simulink model "Previous_Version_2016_b_All_BPF_with_IQ_Demodulation"  (R2020a)
settings: Solver=VariableStepAuto  StartTime=0.0  StopTime=8.2  RelTol=1e-3
libraries: dsphdlxfrm x1
(part 1 of 3)
settings Model: Creator=Renas  LastModifiedBy=Renas

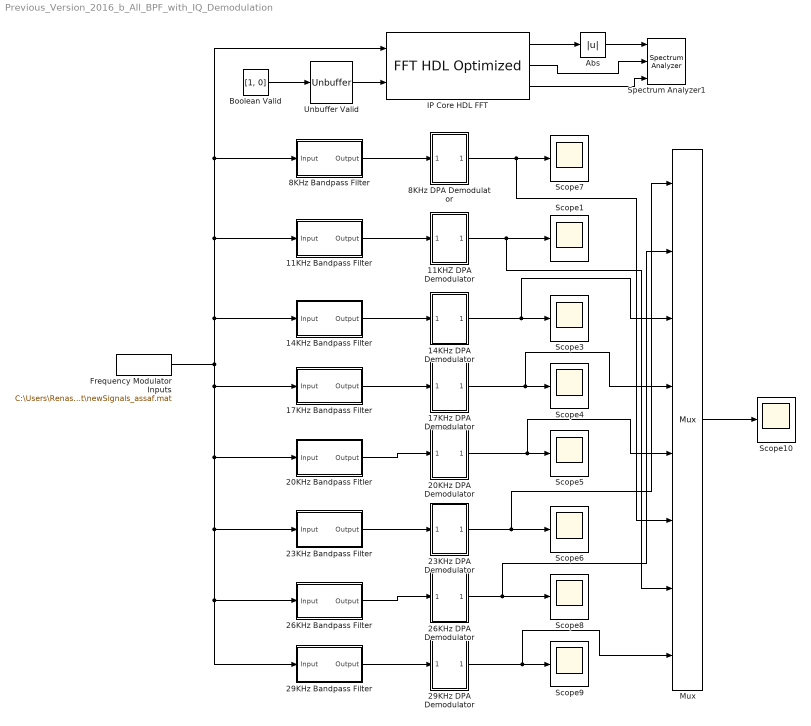
== system Previous_Version_2016_b_All_BPF_with_IQ_Demodulation ==
  11KHZ DPA Demodulator : Subsystem
  11KHz Bandpass Filter : Subsystem  Tag=FilterWizardSubSystem
      settings: ErrorFcn=dspFilterRealizedInBasicElemsAlgLoopErrFcnCallback
  14KHz Bandpass Filter : Subsystem  Tag=FilterWizardSubSystem
      settings: ErrorFcn=dspFilterRealizedInBasicElemsAlgLoopErrFcnCallback
  14KHz DPA Demodulator : Subsystem
  17KHz Bandpass Filter : Subsystem  Tag=FilterWizardSubSystem
      settings: ErrorFcn=dspFilterRealizedInBasicElemsAlgLoopErrFcnCallback
  17KHz DPA Demodulator : Subsystem
  20KHz Bandpass Fitler : Subsystem  Tag=FilterWizardSubSystem
      settings: ErrorFcn=dspFilterRealizedInBasicElemsAlgLoopErrFcnCallback
  20KHz DPA Demodulator : Subsystem
  23KHz Bandpass Filter : Subsystem  Tag=FilterWizardSubSystem
      settings: ErrorFcn=dspFilterRealizedInBasicElemsAlgLoopErrFcnCallback
  23KHz DPA Demodulator : Subsystem
  26KHz Bandpass Filter : Subsystem  Tag=FilterWizardSubSystem
      settings: ErrorFcn=dspFilterRealizedInBasicElemsAlgLoopErrFcnCallback
  26KHz DPA Demodulator : Subsystem
  29KHz Bandpass Filter : Subsystem  Tag=FilterWizardSubSystem
      settings: ErrorFcn=dspFilterRealizedInBasicElemsAlgLoopErrFcnCallback
  29KHz DPA Demodulator : Subsystem
  8KHz Bandpass Filter : Subsystem  Tag=FilterWizardSubSystem
      settings: ErrorFcn=dspFilterRealizedInBasicElemsAlgLoopErrFcnCallback
  8KHz DPA Demodulator : Subsystem
  Abs : Abs
  Boolean Valid : Constant  Value=[1, 0]  OutDataTypeStr=boolean  SampleTime=0.000004
  Frequency Modulator Inputs : FromFile  FileName=C:\Users\Renas\Desktop\Final Year Project\newSignals_assaf.mat  SampleTime=0.000004
  IP Core HDL FFT : dsphdlxfrm/FFT HDL Optimized  FFTLength=8  Architecture=Burst Radix 2  ComplexMultiplication=Use 4 multipliers and 2 adders  BitReversedOutput=off  BitReversedInput=off  Normalize=off  SimulateUsing=Code generation  RoundingMethod=Nearest  ResetInputPort=off  StartOutputPort=off  EndOutputPort=off
      settings: SourceProductBaseCode=DS
  Mux : Mux  Inputs=8
      settings: DisplayOption=signals
  Scope{1,3..10} (9 alike) : Scope
  Spectrum Analyzer1 : SpectrumAnalyzer  NumInputPorts=3
  Unbuffer Valid : Unbuffer
  wires:
  8KHz Bandpass Filter/1(Output) -> 8KHz DPA Demodulator/1(In3)
  11KHZ DPA Demodulator/1(Out1) -> Mux/7, Scope1/1
  11KHz Bandpass Filter/1(Output) -> 11KHZ DPA Demodulator/1(Output)
  14KHz DPA Demodulator/1(Out1) -> Mux/3, Scope3/1
  17KHz DPA Demodulator/1(Out1) -> Scope4/1, Mux/4
  20KHz DPA Demodulator/1(Out1) -> Scope5/1, Mux/5
  23KHz DPA Demodulator/1(Out1) -> Mux/1, Scope6/1
  26KHz DPA Demodulator/1(Out1) -> Mux/2, Scope8/1
  29KHz DPA Demodulator/1(Out1) -> Mux/8, Scope9/1
  Mux/1 -> Scope10/1
  8KHz DPA Demodulator/1(Out1) -> Mux/6, Scope7/1
  14KHz Bandpass Filter/1(Output) -> 14KHz DPA Demodulator/1(Output)
  17KHz Bandpass Filter/1(Output) -> 17KHz DPA Demodulator/1(Output)
  20KHz Bandpass Fitler/1(Output) -> 20KHz DPA Demodulator/1(Output)
  23KHz Bandpass Filter/1(Output) -> 23KHz DPA Demodulator/1(Output)
  26KHz Bandpass Filter/1(Output) -> 26KHz DPA Demodulator/1(Output)
  29KHz Bandpass Filter/1(Output) -> 29KHz DPA Demodulator/1(Output)
  Frequency Modulator Inputs/1 -> IP Core HDL FFT/1, 8KHz Bandpass Filter/1(Input), 11KHz Bandpass Filter/1(Input), 14KHz Bandpass Filter/1(Input), 29KHz Bandpass Filter/1(Input), 26KHz Bandpass Filter/1(Input), 23KHz Bandpass Filter/1(Input), 20KHz Bandpass Fitler/1(Input), 17KHz Bandpass Filter/1(Input)
  IP Core HDL FFT/1 -> Abs/1
  IP Core HDL FFT/3 -> Spectrum Analyzer1/3
  IP Core HDL FFT/2 -> Spectrum Analyzer1/2
  Abs/1 -> Spectrum Analyzer1/1
  Boolean Valid/1 -> Unbuffer Valid/1
  Unbuffer Valid/1 -> IP Core HDL FFT/2

== system Previous_Version_2016_b_All_BPF_with_IQ_Demodulation/11KHZ DPA Demodulator ==
  note: "Imaginary"
  note: "Real"
  Output : Inport
  Delay : Delay  DelayLength=1  InitialCondition=0
  Delay1 : Delay  DelayLength=1  InitialCondition=0
  Divide : Product  Inputs=*/
  Gain1 : Gain  Gain=7.5/((0.000004)*(2*pi*1000))
  Gain2 : Gain  Gain=-1
  LPF_11000Hz_Elliptical_100dB_BW_2KHz_Order_1 : Subsystem  Tag=FilterWizardSubSystem
      settings: ErrorFcn=dspFilterRealizedInBasicElemsAlgLoopErrFcnCallback
  LPF_11000Hz_Elliptical_100dB_BW_2KHz_Order_10 : Subsystem  Tag=FilterWizardSubSystem
      settings: ErrorFcn=dspFilterRealizedInBasicElemsAlgLoopErrFcnCallback
  Product{5..10} (6 alike) : Product
  Scope : Scope
  Scope5 : Scope
  Scope6 : Scope
  Sine Wave : Sin  Frequency=2*pi*11000  Phase=+(pi/2)  Samples=250  SampleTime=1/250000
  Sine Wave1 : Sin  Frequency=2*pi*11000  SampleTime=1/250000
  Sum : Sum  Inputs=|++
  Sum1 : Sum  Inputs=|+-
  Trigonometric Function1 : Trigonometry  Operator=atan
  Out1 : Outport
  wires:
  LPF_11000Hz_Elliptical_100dB_BW_2KHz_Order_10/1(Output) -> Scope5/1, Product10/1, Product9/1, Delay1/1
  Delay/1 -> Product8/1, Product9/2
  Gain2/1 -> Product8/2, Product6/2, Delay/1
  Delay1/1 -> Product6/1, Product10/2
  Divide/1 -> Trigonometric Function1/1
  Gain1/1 -> Out1/1
  Product6/1 -> Sum1/1
  Sum/1 -> Divide/2
  Sum1/1 -> Divide/1
  Product5/1 -> LPF_11000Hz_Elliptical_100dB_BW_2KHz_Order_10/1(Input)
  Product8/1 -> Sum/2
  Product9/1 -> Sum1/2
  Sine Wave1/1 -> Product5/2
  Output/1 -> Product5/1, Product7/2, Scope/1
  LPF_11000Hz_Elliptical_100dB_BW_2KHz_Order_1/1(Output) -> Gain2/1, Scope6/1
  Product10/1 -> Sum/1
  Sine Wave/1 -> Product7/1
  Product7/1 -> LPF_11000Hz_Elliptical_100dB_BW_2KHz_Order_1/1(Input)
  Trigonometric Function1/1 -> Gain1/1

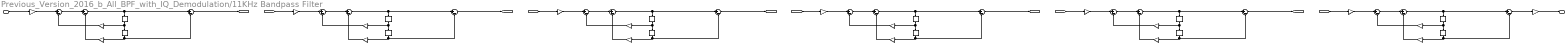
== system Previous_Version_2016_b_All_BPF_with_IQ_Demodulation/11KHz Bandpass Filter ==
  Input : Inport
  Delay{11..16,21..26} (12 alike) : Delay  DelayLength=1  InitialCondition=0
  SumA{21..26,31..36} (12 alike) : Sum  Inputs=|+-  RndMeth=Nearest  SaturateOnIntegerOverflow=on  OutDataTypeStr=Inherit: Same as first input
  SumB{31..36} (6 alike) : Sum  Inputs=|+-  RndMeth=Nearest  SaturateOnIntegerOverflow=on  OutDataTypeStr=Inherit: Same as first input
  a(2)(1) : Gain  Gain=-1.9065952938784374  ParamDataTypeStr=double  RndMeth=Nearest  SaturateOnIntegerOverflow=on  OutDataTypeStr=Inherit: Same as input
  a(2)(2) : Gain  Gain=-1.93433571126361903  ParamDataTypeStr=double  RndMeth=Nearest  SaturateOnIntegerOverflow=on  OutDataTypeStr=Inherit: Same as input
  a(2)(3) : Gain  Gain=-1.90539970784921886  ParamDataTypeStr=double  RndMeth=Nearest  SaturateOnIntegerOverflow=on  OutDataTypeStr=Inherit: Same as input
  a(2)(4) : Gain  Gain=-1.92628834700168183  ParamDataTypeStr=double  RndMeth=Nearest  SaturateOnIntegerOverflow=on  OutDataTypeStr=Inherit: Same as input
  a(2)(5) : Gain  Gain=-1.90953396328044223  ParamDataTypeStr=double  RndMeth=Nearest  SaturateOnIntegerOverflow=on  OutDataTypeStr=Inherit: Same as input
  a(2)(6) : Gain  Gain=-1.91729782266235227  ParamDataTypeStr=double  RndMeth=Nearest  SaturateOnIntegerOverflow=on  OutDataTypeStr=Inherit: Same as input
  a(3)(1) : Gain  Gain=0.996606493218230471  ParamDataTypeStr=double  RndMeth=Nearest  SaturateOnIntegerOverflow=on  OutDataTypeStr=Inherit: Same as input
  a(3)(2) : Gain  Gain=0.997154789899552862  ParamDataTypeStr=double  RndMeth=Nearest  SaturateOnIntegerOverflow=on  OutDataTypeStr=Inherit: Same as input
  a(3)(3) : Gain  Gain=0.990951691511379074  ParamDataTypeStr=double  RndMeth=Nearest  SaturateOnIntegerOverflow=on  OutDataTypeStr=Inherit: Same as input
  a(3)(4) : Gain  Gain=0.992044936946816946  ParamDataTypeStr=double  RndMeth=Nearest  SaturateOnIntegerOverflow=on  OutDataTypeStr=Inherit: Same as input
  a(3)(5) : Gain  Gain=0.988127915993850081  ParamDataTypeStr=double  RndMeth=Nearest  SaturateOnIntegerOverflow=on  OutDataTypeStr=Inherit: Same as input
  a(3)(6) : Gain  Gain=0.98867412178745806  ParamDataTypeStr=double  RndMeth=Nearest  SaturateOnIntegerOverflow=on  OutDataTypeStr=Inherit: Same as input
  s(1) : Gain  Gain=0.0249744654943324963  ParamDataTypeStr=double  RndMeth=Nearest  SaturateOnIntegerOverflow=on  OutDataTypeStr=Inherit: Same as input
  s(2) : Gain  Gain=0.0249744654943324963  ParamDataTypeStr=double  RndMeth=Nearest  SaturateOnIntegerOverflow=on  OutDataTypeStr=Inherit: Same as input
  s(3) : Gain  Gain=0.0186903150291070699  ParamDataTypeStr=double  RndMeth=Nearest  SaturateOnIntegerOverflow=on  OutDataTypeStr=Inherit: Same as input
  s(4) : Gain  Gain=0.0186903150291070699  ParamDataTypeStr=double  RndMeth=Nearest  SaturateOnIntegerOverflow=on  OutDataTypeStr=Inherit: Same as input
  s(5) : Gain  Gain=0.00882552998553000692  ParamDataTypeStr=double  RndMeth=Nearest  SaturateOnIntegerOverflow=on  OutDataTypeStr=Inherit: Same as input
  s(6) : Gain  Gain=0.00882552998553000692  ParamDataTypeStr=double  RndMeth=Nearest  SaturateOnIntegerOverflow=on  OutDataTypeStr=Inherit: Same as input
  s(7) : Gain  Gain=0.891250938133745563  ParamDataTypeStr=double  RndMeth=Nearest  SaturateOnIntegerOverflow=on  OutDataTypeStr=Inherit: Same as input
  Output : Outport
  wires:
  Input/1 -> s(1)/1
  s(1)/1 -> SumA21/1
  SumA21/1 -> SumA31/1
  SumA31/1 -> SumB31/1, Delay11/1
  SumB31/1 -> [Sect1]
  a(2)(1)/1 -> SumA21/2
  Delay11/1 -> a(2)(1)/1, Delay21/1
  a(3)(1)/1 -> SumA31/2
  Delay21/1 -> a(3)(1)/1, SumB31/2
  [Sect1] -> s(2)/1
  s(2)/1 -> SumA22/1
  SumA22/1 -> SumA32/1
  SumA32/1 -> SumB32/1, Delay12/1
  SumB32/1 -> [Sect2]
  a(2)(2)/1 -> SumA22/2
  Delay12/1 -> a(2)(2)/1, Delay22/1
  a(3)(2)/1 -> SumA32/2
  Delay22/1 -> a(3)(2)/1, SumB32/2
  [Sect2] -> s(3)/1
  s(3)/1 -> SumA23/1
  SumA23/1 -> SumA33/1
  SumA33/1 -> SumB33/1, Delay13/1
  SumB33/1 -> [Sect3]
  a(2)(3)/1 -> SumA23/2
  Delay13/1 -> a(2)(3)/1, Delay23/1
  a(3)(3)/1 -> SumA33/2
  Delay23/1 -> a(3)(3)/1, SumB33/2
  [Sect3] -> s(4)/1
  s(4)/1 -> SumA24/1
  SumA24/1 -> SumA34/1
  SumA34/1 -> SumB34/1, Delay14/1
  SumB34/1 -> [Sect4]
  a(2)(4)/1 -> SumA24/2
  Delay14/1 -> a(2)(4)/1, Delay24/1
  a(3)(4)/1 -> SumA34/2
  Delay24/1 -> a(3)(4)/1, SumB34/2
  [Sect4] -> s(5)/1
  s(5)/1 -> SumA25/1
  SumA25/1 -> SumA35/1
  SumA35/1 -> SumB35/1, Delay15/1
  SumB35/1 -> [Sect5]
  a(2)(5)/1 -> SumA25/2
  Delay15/1 -> a(2)(5)/1, Delay25/1
  a(3)(5)/1 -> SumA35/2
  Delay25/1 -> a(3)(5)/1, SumB35/2
  [Sect5] -> s(6)/1
  s(6)/1 -> SumA26/1
  SumA26/1 -> SumA36/1
  SumA36/1 -> SumB36/1, Delay16/1
  SumB36/1 -> s(7)/1
  a(2)(6)/1 -> SumA26/2
  Delay16/1 -> a(2)(6)/1, Delay26/1
  a(3)(6)/1 -> SumA36/2
  Delay26/1 -> a(3)(6)/1, SumB36/2
  s(7)/1 -> Output/1

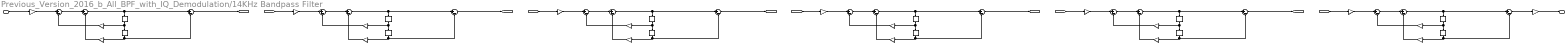
== system Previous_Version_2016_b_All_BPF_with_IQ_Demodulation/14KHz Bandpass Filter ==
  Input : Inport
  Delay{11..16,21..26} (12 alike) : Delay  DelayLength=1  InitialCondition=0
  SumA{21..26,31..36} (12 alike) : Sum  Inputs=|+-  RndMeth=Nearest  SaturateOnIntegerOverflow=on  OutDataTypeStr=Inherit: Same as first input
  SumB{31..36} (6 alike) : Sum  Inputs=|+-  RndMeth=Nearest  SaturateOnIntegerOverflow=on  OutDataTypeStr=Inherit: Same as first input
  a(2)(1) : Gain  Gain=-1.85547628075388515  ParamDataTypeStr=double  RndMeth=Nearest  SaturateOnIntegerOverflow=on  OutDataTypeStr=Inherit: Same as input
  a(2)(2) : Gain  Gain=-1.89037409301842607  ParamDataTypeStr=double  RndMeth=Nearest  SaturateOnIntegerOverflow=on  OutDataTypeStr=Inherit: Same as input
  a(2)(3) : Gain  Gain=-1.85544003350902065  ParamDataTypeStr=double  RndMeth=Nearest  SaturateOnIntegerOverflow=on  OutDataTypeStr=Inherit: Same as input
  a(2)(4) : Gain  Gain=-1.88139619531860136  ParamDataTypeStr=double  RndMeth=Nearest  SaturateOnIntegerOverflow=on  OutDataTypeStr=Inherit: Same as input
  a(2)(5) : Gain  Gain=-1.86125831898491256  ParamDataTypeStr=double  RndMeth=Nearest  SaturateOnIntegerOverflow=on  OutDataTypeStr=Inherit: Same as input
  a(2)(6) : Gain  Gain=-1.87084185582867502  ParamDataTypeStr=double  RndMeth=Nearest  SaturateOnIntegerOverflow=on  OutDataTypeStr=Inherit: Same as input
  a(3)(1) : Gain  Gain=0.996669751260965242  ParamDataTypeStr=double  RndMeth=Nearest  SaturateOnIntegerOverflow=on  OutDataTypeStr=Inherit: Same as input
  a(3)(2) : Gain  Gain=0.997091501071703412  ParamDataTypeStr=double  RndMeth=Nearest  SaturateOnIntegerOverflow=on  OutDataTypeStr=Inherit: Same as input
  a(3)(3) : Gain  Gain=0.991078116538709697  ParamDataTypeStr=double  RndMeth=Nearest  SaturateOnIntegerOverflow=on  OutDataTypeStr=Inherit: Same as input
  a(3)(4) : Gain  Gain=0.991918388588846511  ParamDataTypeStr=double  RndMeth=Nearest  SaturateOnIntegerOverflow=on  OutDataTypeStr=Inherit: Same as input
  a(3)(5) : Gain  Gain=0.988191259658187882  ParamDataTypeStr=double  RndMeth=Nearest  SaturateOnIntegerOverflow=on  OutDataTypeStr=Inherit: Same as input
  a(3)(6) : Gain  Gain=0.988610747171366766  ParamDataTypeStr=double  RndMeth=Nearest  SaturateOnIntegerOverflow=on  OutDataTypeStr=Inherit: Same as input
  s(1) : Gain  Gain=0.0249744654943327288  ParamDataTypeStr=double  RndMeth=Nearest  SaturateOnIntegerOverflow=on  OutDataTypeStr=Inherit: Same as input
  s(2) : Gain  Gain=0.0249744654943327288  ParamDataTypeStr=double  RndMeth=Nearest  SaturateOnIntegerOverflow=on  OutDataTypeStr=Inherit: Same as input
  s(3) : Gain  Gain=0.0186903150291072434  ParamDataTypeStr=double  RndMeth=Nearest  SaturateOnIntegerOverflow=on  OutDataTypeStr=Inherit: Same as input
  s(4) : Gain  Gain=0.0186903150291072434  ParamDataTypeStr=double  RndMeth=Nearest  SaturateOnIntegerOverflow=on  OutDataTypeStr=Inherit: Same as input
  s(5) : Gain  Gain=0.00882552998553009019  ParamDataTypeStr=double  RndMeth=Nearest  SaturateOnIntegerOverflow=on  OutDataTypeStr=Inherit: Same as input
  s(6) : Gain  Gain=0.00882552998553009019  ParamDataTypeStr=double  RndMeth=Nearest  SaturateOnIntegerOverflow=on  OutDataTypeStr=Inherit: Same as input
  s(7) : Gain  Gain=0.891250938133745563  ParamDataTypeStr=double  RndMeth=Nearest  SaturateOnIntegerOverflow=on  OutDataTypeStr=Inherit: Same as input
  Output : Outport
  wires:
  Input/1 -> s(1)/1
  s(1)/1 -> SumA21/1
  SumA21/1 -> SumA31/1
  SumA31/1 -> SumB31/1, Delay11/1
  SumB31/1 -> [Sect1]
  a(2)(1)/1 -> SumA21/2
  Delay11/1 -> a(2)(1)/1, Delay21/1
  a(3)(1)/1 -> SumA31/2
  Delay21/1 -> a(3)(1)/1, SumB31/2
  [Sect1] -> s(2)/1
  s(2)/1 -> SumA22/1
  SumA22/1 -> SumA32/1
  SumA32/1 -> SumB32/1, Delay12/1
  SumB32/1 -> [Sect2]
  a(2)(2)/1 -> SumA22/2
  Delay12/1 -> a(2)(2)/1, Delay22/1
  a(3)(2)/1 -> SumA32/2
  Delay22/1 -> a(3)(2)/1, SumB32/2
  [Sect2] -> s(3)/1
  s(3)/1 -> SumA23/1
  SumA23/1 -> SumA33/1
  SumA33/1 -> SumB33/1, Delay13/1
  SumB33/1 -> [Sect3]
  a(2)(3)/1 -> SumA23/2
  Delay13/1 -> a(2)(3)/1, Delay23/1
  a(3)(3)/1 -> SumA33/2
  Delay23/1 -> a(3)(3)/1, SumB33/2
  [Sect3] -> s(4)/1
  s(4)/1 -> SumA24/1
  SumA24/1 -> SumA34/1
  SumA34/1 -> SumB34/1, Delay14/1
  SumB34/1 -> [Sect4]
  a(2)(4)/1 -> SumA24/2
  Delay14/1 -> a(2)(4)/1, Delay24/1
  a(3)(4)/1 -> SumA34/2
  Delay24/1 -> a(3)(4)/1, SumB34/2
  [Sect4] -> s(5)/1
  s(5)/1 -> SumA25/1
  SumA25/1 -> SumA35/1
  SumA35/1 -> SumB35/1, Delay15/1
  SumB35/1 -> [Sect5]
  a(2)(5)/1 -> SumA25/2
  Delay15/1 -> a(2)(5)/1, Delay25/1
  a(3)(5)/1 -> SumA35/2
  Delay25/1 -> a(3)(5)/1, SumB35/2
  [Sect5] -> s(6)/1
  s(6)/1 -> SumA26/1
  SumA26/1 -> SumA36/1
  SumA36/1 -> SumB36/1, Delay16/1
  SumB36/1 -> s(7)/1
  a(2)(6)/1 -> SumA26/2
  Delay16/1 -> a(2)(6)/1, Delay26/1
  a(3)(6)/1 -> SumA36/2
  Delay26/1 -> a(3)(6)/1, SumB36/2
  s(7)/1 -> Output/1

== system Previous_Version_2016_b_All_BPF_with_IQ_Demodulation/14KHz DPA Demodulator ==
  note: "Imaginary"
  note: "Real"
  Output : Inport
  Delay : Delay  DelayLength=1  InitialCondition=0
  Delay1 : Delay  DelayLength=1  InitialCondition=0
  Divide : Product  Inputs=*/
  Gain1 : Gain  Gain=7.5/((0.000004)*(2*pi*1000))
  Gain2 : Gain  Gain=-1
  LPF_14060Hz_Elliptical_100dB_BW_2KHz_Order_1 : Subsystem  Tag=FilterWizardSubSystem
      settings: ErrorFcn=dspFilterRealizedInBasicElemsAlgLoopErrFcnCallback
  LPF_14060Hz_Elliptical_100dB_BW_2KHz_Order_10 : Subsystem  Tag=FilterWizardSubSystem
      settings: ErrorFcn=dspFilterRealizedInBasicElemsAlgLoopErrFcnCallback
  Product{5..10} (6 alike) : Product
  Scope : Scope
  Scope5 : Scope
  Scope6 : Scope
  Sine Wave : Sin  Frequency=2*pi*14060  Phase=+(pi/2)  Samples=250  SampleTime=1/250000
  Sine Wave1 : Sin  Frequency=2*pi*14060  SampleTime=1/250000
  Sum : Sum  Inputs=|++
  Sum1 : Sum  Inputs=|+-
  Trigonometric Function1 : Trigonometry  Operator=atan
  Out1 : Outport
  wires:
  LPF_14060Hz_Elliptical_100dB_BW_2KHz_Order_10/1(Output) -> Scope5/1, Product10/1, Product9/1, Delay1/1
  Delay/1 -> Product8/1, Product9/2
  Gain2/1 -> Product8/2, Product6/2, Delay/1
  Delay1/1 -> Product6/1, Product10/2
  Divide/1 -> Trigonometric Function1/1
  Gain1/1 -> Out1/1
  Product6/1 -> Sum1/1
  Sum/1 -> Divide/2
  Sum1/1 -> Divide/1
  Product5/1 -> LPF_14060Hz_Elliptical_100dB_BW_2KHz_Order_10/1(Input)
  Product8/1 -> Sum/2
  Product9/1 -> Sum1/2
  Sine Wave1/1 -> Product5/2
  Output/1 -> Product5/1, Product7/2, Scope/1
  LPF_14060Hz_Elliptical_100dB_BW_2KHz_Order_1/1(Output) -> Gain2/1, Scope6/1
  Product10/1 -> Sum/1
  Sine Wave/1 -> Product7/1
  Product7/1 -> LPF_14060Hz_Elliptical_100dB_BW_2KHz_Order_1/1(Input)
  Trigonometric Function1/1 -> Gain1/1

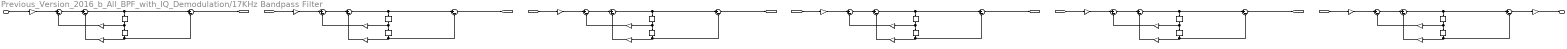
== system Previous_Version_2016_b_All_BPF_with_IQ_Demodulation/17KHz Bandpass Filter ==
  Input : Inport
  Delay{11..16,21..26} (12 alike) : Delay  DelayLength=1  InitialCondition=0
  SumA{21..26,31..36} (12 alike) : Sum  Inputs=|+-  RndMeth=Nearest  SaturateOnIntegerOverflow=on  OutDataTypeStr=Inherit: Same as first input
  SumB{31..36} (6 alike) : Sum  Inputs=|+-  RndMeth=Nearest  SaturateOnIntegerOverflow=on  OutDataTypeStr=Inherit: Same as first input
  a(2)(1) : Gain  Gain=-1.79490617474365566  ParamDataTypeStr=double  RndMeth=Nearest  SaturateOnIntegerOverflow=on  OutDataTypeStr=Inherit: Same as input
  a(2)(2) : Gain  Gain=-1.83664366102072707  ParamDataTypeStr=double  RndMeth=Nearest  SaturateOnIntegerOverflow=on  OutDataTypeStr=Inherit: Same as input
  a(2)(3) : Gain  Gain=-1.79598178570065503  ParamDataTypeStr=double  RndMeth=Nearest  SaturateOnIntegerOverflow=on  OutDataTypeStr=Inherit: Same as input
  a(2)(4) : Gain  Gain=-1.82682896191897925  ParamDataTypeStr=double  RndMeth=Nearest  SaturateOnIntegerOverflow=on  OutDataTypeStr=Inherit: Same as input
  a(2)(5) : Gain  Gain=-1.80343450281448359  ParamDataTypeStr=double  RndMeth=Nearest  SaturateOnIntegerOverflow=on  OutDataTypeStr=Inherit: Same as input
  a(2)(6) : Gain  Gain=-1.81478470631303734  ParamDataTypeStr=double  RndMeth=Nearest  SaturateOnIntegerOverflow=on  OutDataTypeStr=Inherit: Same as input
  a(3)(1) : Gain  Gain=0.996710356003254083  ParamDataTypeStr=double  RndMeth=Nearest  SaturateOnIntegerOverflow=on  OutDataTypeStr=Inherit: Same as input
  a(3)(2) : Gain  Gain=0.997050880802035189  ParamDataTypeStr=double  RndMeth=Nearest  SaturateOnIntegerOverflow=on  OutDataTypeStr=Inherit: Same as input
  a(3)(3) : Gain  Gain=0.991159132334594517  ParamDataTypeStr=double  RndMeth=Nearest  SaturateOnIntegerOverflow=on  OutDataTypeStr=Inherit: Same as input
  a(3)(4) : Gain  Gain=0.991837310732544997  ParamDataTypeStr=double  RndMeth=Nearest  SaturateOnIntegerOverflow=on  OutDataTypeStr=Inherit: Same as input
  a(3)(5) : Gain  Gain=0.988231779244872266  ParamDataTypeStr=double  RndMeth=Nearest  SaturateOnIntegerOverflow=on  OutDataTypeStr=Inherit: Same as input
  a(3)(6) : Gain  Gain=0.988570212046192665  ParamDataTypeStr=double  RndMeth=Nearest  SaturateOnIntegerOverflow=on  OutDataTypeStr=Inherit: Same as input
  s(1) : Gain  Gain=0.0249744654943329404  ParamDataTypeStr=double  RndMeth=Nearest  SaturateOnIntegerOverflow=on  OutDataTypeStr=Inherit: Same as input
  s(2) : Gain  Gain=0.0249744654943329404  ParamDataTypeStr=double  RndMeth=Nearest  SaturateOnIntegerOverflow=on  OutDataTypeStr=Inherit: Same as input
  s(3) : Gain  Gain=0.018690315029107403  ParamDataTypeStr=double  RndMeth=Nearest  SaturateOnIntegerOverflow=on  OutDataTypeStr=Inherit: Same as input
  s(4) : Gain  Gain=0.018690315029107403  ParamDataTypeStr=double  RndMeth=Nearest  SaturateOnIntegerOverflow=on  OutDataTypeStr=Inherit: Same as input
  s(5) : Gain  Gain=0.00882552998553016305  ParamDataTypeStr=double  RndMeth=Nearest  SaturateOnIntegerOverflow=on  OutDataTypeStr=Inherit: Same as input
  s(6) : Gain  Gain=0.00882552998553016305  ParamDataTypeStr=double  RndMeth=Nearest  SaturateOnIntegerOverflow=on  OutDataTypeStr=Inherit: Same as input
  s(7) : Gain  Gain=0.891250938133745563  ParamDataTypeStr=double  RndMeth=Nearest  SaturateOnIntegerOverflow=on  OutDataTypeStr=Inherit: Same as input
  Output : Outport
  wires:
  Input/1 -> s(1)/1
  s(1)/1 -> SumA21/1
  SumA21/1 -> SumA31/1
  SumA31/1 -> SumB31/1, Delay11/1
  SumB31/1 -> [Sect1]
  a(2)(1)/1 -> SumA21/2
  Delay11/1 -> a(2)(1)/1, Delay21/1
  a(3)(1)/1 -> SumA31/2
  Delay21/1 -> a(3)(1)/1, SumB31/2
  [Sect1] -> s(2)/1
  s(2)/1 -> SumA22/1
  SumA22/1 -> SumA32/1
  SumA32/1 -> SumB32/1, Delay12/1
  SumB32/1 -> [Sect2]
  a(2)(2)/1 -> SumA22/2
  Delay12/1 -> a(2)(2)/1, Delay22/1
  a(3)(2)/1 -> SumA32/2
  Delay22/1 -> a(3)(2)/1, SumB32/2
  [Sect2] -> s(3)/1
  s(3)/1 -> SumA23/1
  SumA23/1 -> SumA33/1
  SumA33/1 -> SumB33/1, Delay13/1
  SumB33/1 -> [Sect3]
  a(2)(3)/1 -> SumA23/2
  Delay13/1 -> a(2)(3)/1, Delay23/1
  a(3)(3)/1 -> SumA33/2
  Delay23/1 -> a(3)(3)/1, SumB33/2
  [Sect3] -> s(4)/1
  s(4)/1 -> SumA24/1
  SumA24/1 -> SumA34/1
  SumA34/1 -> SumB34/1, Delay14/1
  SumB34/1 -> [Sect4]
  a(2)(4)/1 -> SumA24/2
  Delay14/1 -> a(2)(4)/1, Delay24/1
  a(3)(4)/1 -> SumA34/2
  Delay24/1 -> a(3)(4)/1, SumB34/2
  [Sect4] -> s(5)/1
  s(5)/1 -> SumA25/1
  SumA25/1 -> SumA35/1
  SumA35/1 -> SumB35/1, Delay15/1
  SumB35/1 -> [Sect5]
  a(2)(5)/1 -> SumA25/2
  Delay15/1 -> a(2)(5)/1, Delay25/1
  a(3)(5)/1 -> SumA35/2
  Delay25/1 -> a(3)(5)/1, SumB35/2
  [Sect5] -> s(6)/1
  s(6)/1 -> SumA26/1
  SumA26/1 -> SumA36/1
  SumA36/1 -> SumB36/1, Delay16/1
  SumB36/1 -> s(7)/1
  a(2)(6)/1 -> SumA26/2
  Delay16/1 -> a(2)(6)/1, Delay26/1
  a(3)(6)/1 -> SumA36/2
  Delay26/1 -> a(3)(6)/1, SumB36/2
  s(7)/1 -> Output/1

== system Previous_Version_2016_b_All_BPF_with_IQ_Demodulation/17KHz DPA Demodulator ==
  note: "Imaginary"
  note: "Real"
  Output : Inport
  Delay : Delay  DelayLength=1  InitialCondition=0
  Delay1 : Delay  DelayLength=1  InitialCondition=0
  Divide : Product  Inputs=*/
  Gain1 : Gain  Gain=7.5/((0.000004)*(2*pi*1000))
  Gain2 : Gain  Gain=-1
  LPF_17050Hz_Elliptical_100dB_BW_2KHz_Order_1 : Subsystem  Tag=FilterWizardSubSystem
      settings: ErrorFcn=dspFilterRealizedInBasicElemsAlgLoopErrFcnCallback
  LPF_17050Hz_Elliptical_100dB_BW_2KHz_Order_10 : Subsystem  Tag=FilterWizardSubSystem
      settings: ErrorFcn=dspFilterRealizedInBasicElemsAlgLoopErrFcnCallback
  Product{5..10} (6 alike) : Product
  Scope : Scope
  Scope5 : Scope
  Scope6 : Scope
  Sine Wave : Sin  Frequency=2*pi*17050  Phase=+(pi/2)  Samples=250  SampleTime=1/250000
  Sine Wave1 : Sin  Frequency=2*pi*17050  SampleTime=1/250000
  Sum : Sum  Inputs=|++
  Sum1 : Sum  Inputs=|+-
  Trigonometric Function1 : Trigonometry  Operator=atan
  Out1 : Outport
  wires:
  LPF_17050Hz_Elliptical_100dB_BW_2KHz_Order_10/1(Output) -> Scope5/1, Product10/1, Product9/1, Delay1/1
  Delay/1 -> Product8/1, Product9/2
  Gain2/1 -> Product8/2, Product6/2, Delay/1
  Delay1/1 -> Product6/1, Product10/2
  Divide/1 -> Trigonometric Function1/1
  Gain1/1 -> Out1/1
  Product6/1 -> Sum1/1
  Sum/1 -> Divide/2
  Sum1/1 -> Divide/1
  Product5/1 -> LPF_17050Hz_Elliptical_100dB_BW_2KHz_Order_10/1(Input)
  Product8/1 -> Sum/2
  Product9/1 -> Sum1/2
  Sine Wave1/1 -> Product5/2
  Output/1 -> Product5/1, Product7/2, Scope/1
  LPF_17050Hz_Elliptical_100dB_BW_2KHz_Order_1/1(Output) -> Gain2/1, Scope6/1
  Product10/1 -> Sum/1
  Sine Wave/1 -> Product7/1
  Product7/1 -> LPF_17050Hz_Elliptical_100dB_BW_2KHz_Order_1/1(Input)
  Trigonometric Function1/1 -> Gain1/1

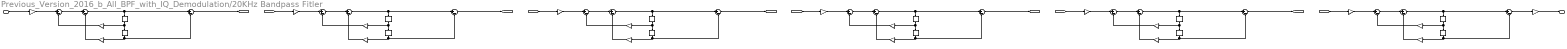
== system Previous_Version_2016_b_All_BPF_with_IQ_Demodulation/20KHz Bandpass Fitler ==
  Input : Inport
  Delay{11..16,21..26} (12 alike) : Delay  DelayLength=1  InitialCondition=0
  SumA{21..26,31..36} (12 alike) : Sum  Inputs=|+-  RndMeth=Nearest  SaturateOnIntegerOverflow=on  OutDataTypeStr=Inherit: Same as first input
  SumB{31..36} (6 alike) : Sum  Inputs=|+-  RndMeth=Nearest  SaturateOnIntegerOverflow=on  OutDataTypeStr=Inherit: Same as first input
  a(2)(1) : Gain  Gain=-1.72621306906651273  ParamDataTypeStr=double  RndMeth=Nearest  SaturateOnIntegerOverflow=on  OutDataTypeStr=Inherit: Same as input
  a(2)(2) : Gain  Gain=-1.77440557550816225  ParamDataTypeStr=double  RndMeth=Nearest  SaturateOnIntegerOverflow=on  OutDataTypeStr=Inherit: Same as input
  a(2)(3) : Gain  Gain=-1.72835364533195657  ParamDataTypeStr=double  RndMeth=Nearest  SaturateOnIntegerOverflow=on  OutDataTypeStr=Inherit: Same as input
  a(2)(4) : Gain  Gain=-1.76384098848158066  ParamDataTypeStr=double  RndMeth=Nearest  SaturateOnIntegerOverflow=on  OutDataTypeStr=Inherit: Same as input
  a(2)(5) : Gain  Gain=-1.73736864335266916  ParamDataTypeStr=double  RndMeth=Nearest  SaturateOnIntegerOverflow=on  OutDataTypeStr=Inherit: Same as input
  a(2)(6) : Gain  Gain=-1.75039999440418348  ParamDataTypeStr=double  RndMeth=Nearest  SaturateOnIntegerOverflow=on  OutDataTypeStr=Inherit: Same as input
  a(3)(1) : Gain  Gain=0.996738796712808406  ParamDataTypeStr=double  RndMeth=Nearest  SaturateOnIntegerOverflow=on  OutDataTypeStr=Inherit: Same as input
  a(3)(2) : Gain  Gain=0.997022431187548186  ParamDataTypeStr=double  RndMeth=Nearest  SaturateOnIntegerOverflow=on  OutDataTypeStr=Inherit: Same as input
  a(3)(3) : Gain  Gain=0.991215828337085325  ParamDataTypeStr=double  RndMeth=Nearest  SaturateOnIntegerOverflow=on  OutDataTypeStr=Inherit: Same as input
  a(3)(4) : Gain  Gain=0.991780579182228283  ParamDataTypeStr=double  RndMeth=Nearest  SaturateOnIntegerOverflow=on  OutDataTypeStr=Inherit: Same as input
  a(3)(5) : Gain  Gain=0.988260108481855859  ParamDataTypeStr=double  RndMeth=Nearest  SaturateOnIntegerOverflow=on  OutDataTypeStr=Inherit: Same as input
  a(3)(6) : Gain  Gain=0.988541873919856595  ParamDataTypeStr=double  RndMeth=Nearest  SaturateOnIntegerOverflow=on  OutDataTypeStr=Inherit: Same as input
  s(1) : Gain  Gain=0.0249744654943329925  ParamDataTypeStr=double  RndMeth=Nearest  SaturateOnIntegerOverflow=on  OutDataTypeStr=Inherit: Same as input
  s(2) : Gain  Gain=0.0249744654943329925  ParamDataTypeStr=double  RndMeth=Nearest  SaturateOnIntegerOverflow=on  OutDataTypeStr=Inherit: Same as input
  s(3) : Gain  Gain=0.0186903150291074446  ParamDataTypeStr=double  RndMeth=Nearest  SaturateOnIntegerOverflow=on  OutDataTypeStr=Inherit: Same as input
  s(4) : Gain  Gain=0.0186903150291074446  ParamDataTypeStr=double  RndMeth=Nearest  SaturateOnIntegerOverflow=on  OutDataTypeStr=Inherit: Same as input
  s(5) : Gain  Gain=0.00882552998553018213  ParamDataTypeStr=double  RndMeth=Nearest  SaturateOnIntegerOverflow=on  OutDataTypeStr=Inherit: Same as input
  s(6) : Gain  Gain=0.00882552998553018213  ParamDataTypeStr=double  RndMeth=Nearest  SaturateOnIntegerOverflow=on  OutDataTypeStr=Inherit: Same as input
  s(7) : Gain  Gain=0.891250938133745563  ParamDataTypeStr=double  RndMeth=Nearest  SaturateOnIntegerOverflow=on  OutDataTypeStr=Inherit: Same as input
  Output : Outport
  wires:
  Input/1 -> s(1)/1
  s(1)/1 -> SumA21/1
  SumA21/1 -> SumA31/1
  SumA31/1 -> SumB31/1, Delay11/1
  SumB31/1 -> [Sect1]
  a(2)(1)/1 -> SumA21/2
  Delay11/1 -> a(2)(1)/1, Delay21/1
  a(3)(1)/1 -> SumA31/2
  Delay21/1 -> a(3)(1)/1, SumB31/2
  [Sect1] -> s(2)/1
  s(2)/1 -> SumA22/1
  SumA22/1 -> SumA32/1
  SumA32/1 -> SumB32/1, Delay12/1
  SumB32/1 -> [Sect2]
  a(2)(2)/1 -> SumA22/2
  Delay12/1 -> a(2)(2)/1, Delay22/1
  a(3)(2)/1 -> SumA32/2
  Delay22/1 -> a(3)(2)/1, SumB32/2
  [Sect2] -> s(3)/1
  s(3)/1 -> SumA23/1
  SumA23/1 -> SumA33/1
  SumA33/1 -> SumB33/1, Delay13/1
  SumB33/1 -> [Sect3]
  a(2)(3)/1 -> SumA23/2
  Delay13/1 -> a(2)(3)/1, Delay23/1
  a(3)(3)/1 -> SumA33/2
  Delay23/1 -> a(3)(3)/1, SumB33/2
  [Sect3] -> s(4)/1
  s(4)/1 -> SumA24/1
  SumA24/1 -> SumA34/1
  SumA34/1 -> SumB34/1, Delay14/1
  SumB34/1 -> [Sect4]
  a(2)(4)/1 -> SumA24/2
  Delay14/1 -> a(2)(4)/1, Delay24/1
  a(3)(4)/1 -> SumA34/2
  Delay24/1 -> a(3)(4)/1, SumB34/2
  [Sect4] -> s(5)/1
  s(5)/1 -> SumA25/1
  SumA25/1 -> SumA35/1
  SumA35/1 -> SumB35/1, Delay15/1
  SumB35/1 -> [Sect5]
  a(2)(5)/1 -> SumA25/2
  Delay15/1 -> a(2)(5)/1, Delay25/1
  a(3)(5)/1 -> SumA35/2
  Delay25/1 -> a(3)(5)/1, SumB35/2
  [Sect5] -> s(6)/1
  s(6)/1 -> SumA26/1
  SumA26/1 -> SumA36/1
  SumA36/1 -> SumB36/1, Delay16/1
  SumB36/1 -> s(7)/1
  a(2)(6)/1 -> SumA26/2
  Delay16/1 -> a(2)(6)/1, Delay26/1
  a(3)(6)/1 -> SumA36/2
  Delay26/1 -> a(3)(6)/1, SumB36/2
  s(7)/1 -> Output/1

== system Previous_Version_2016_b_All_BPF_with_IQ_Demodulation/20KHz DPA Demodulator ==
  note: "Imaginary"
  note: "Real"
  Output : Inport
  Delay : Delay  DelayLength=1  InitialCondition=0
  Delay1 : Delay  DelayLength=1  InitialCondition=0
  Divide : Product  Inputs=*/
  Gain1 : Gain  Gain=7.5/((0.000004)*(2*pi*1000))
  Gain2 : Gain  Gain=-1
  LPF_19960Hz_Elliptical_100dB_BW_2KHz_Order_1 : Subsystem  Tag=FilterWizardSubSystem
      settings: ErrorFcn=dspFilterRealizedInBasicElemsAlgLoopErrFcnCallback
  LPF_19960Hz_Elliptical_100dB_BW_2KHz_Order_10 : Subsystem  Tag=FilterWizardSubSystem
      settings: ErrorFcn=dspFilterRealizedInBasicElemsAlgLoopErrFcnCallback
  Product{5..10} (6 alike) : Product
  Scope : Scope
  Scope5 : Scope
  Scope6 : Scope
  Sine Wave : Sin  Frequency=2*pi*19960  Phase=+(pi/2)  Samples=250  SampleTime=1/250000
  Sine Wave1 : Sin  Frequency=2*pi*19960  SampleTime=1/250000
  Sum : Sum  Inputs=|++
  Sum1 : Sum  Inputs=|+-
  Trigonometric Function1 : Trigonometry  Operator=atan
  Out1 : Outport
  wires:
  LPF_19960Hz_Elliptical_100dB_BW_2KHz_Order_10/1(Output) -> Scope5/1, Product10/1, Product9/1, Delay1/1
  Delay/1 -> Product8/1, Product9/2
  Gain2/1 -> Product8/2, Product6/2, Delay/1
  Delay1/1 -> Product6/1, Product10/2
  Divide/1 -> Trigonometric Function1/1
  Gain1/1 -> Out1/1
  Product6/1 -> Sum1/1
  Sum/1 -> Divide/2
  Sum1/1 -> Divide/1
  Product5/1 -> LPF_19960Hz_Elliptical_100dB_BW_2KHz_Order_10/1(Input)
  Product8/1 -> Sum/2
  Product9/1 -> Sum1/2
  Sine Wave1/1 -> Product5/2
  Output/1 -> Product5/1, Product7/2, Scope/1
  LPF_19960Hz_Elliptical_100dB_BW_2KHz_Order_1/1(Output) -> Gain2/1, Scope6/1
  Product10/1 -> Sum/1
  Sine Wave/1 -> Product7/1
  Product7/1 -> LPF_19960Hz_Elliptical_100dB_BW_2KHz_Order_1/1(Input)
  Trigonometric Function1/1 -> Gain1/1

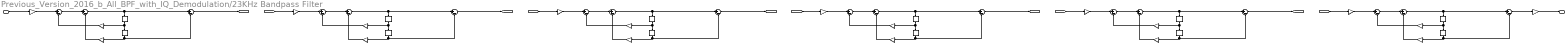
== system Previous_Version_2016_b_All_BPF_with_IQ_Demodulation/23KHz Bandpass Filter ==
  Input : Inport
  Delay{11..16,21..26} (12 alike) : Delay  DelayLength=1  InitialCondition=0
  SumA{21..26,31..36} (12 alike) : Sum  Inputs=|+-  RndMeth=Nearest  SaturateOnIntegerOverflow=on  OutDataTypeStr=Inherit: Same as first input
  SumB{31..36} (6 alike) : Sum  Inputs=|+-  RndMeth=Nearest  SaturateOnIntegerOverflow=on  OutDataTypeStr=Inherit: Same as first input
  a(2)(1) : Gain  Gain=-1.64231285528152715  ParamDataTypeStr=double  RndMeth=Nearest  SaturateOnIntegerOverflow=on  OutDataTypeStr=Inherit: Same as input
  a(2)(2) : Gain  Gain=-1.69715585214219788  ParamDataTypeStr=double  RndMeth=Nearest  SaturateOnIntegerOverflow=on  OutDataTypeStr=Inherit: Same as input
  a(2)(3) : Gain  Gain=-1.64557454783664148  ParamDataTypeStr=double  RndMeth=Nearest  SaturateOnIntegerOverflow=on  OutDataTypeStr=Inherit: Same as input
  a(2)(4) : Gain  Gain=-1.68585794565346614  ParamDataTypeStr=double  RndMeth=Nearest  SaturateOnIntegerOverflow=on  OutDataTypeStr=Inherit: Same as input
  a(2)(5) : Gain  Gain=-1.65621903578087482  ParamDataTypeStr=double  RndMeth=Nearest  SaturateOnIntegerOverflow=on  OutDataTypeStr=Inherit: Same as input
  a(2)(6) : Gain  Gain=-1.67099121106337112  ParamDataTypeStr=double  RndMeth=Nearest  SaturateOnIntegerOverflow=on  OutDataTypeStr=Inherit: Same as input
  a(3)(1) : Gain  Gain=0.996761911818565771  ParamDataTypeStr=double  RndMeth=Nearest  SaturateOnIntegerOverflow=on  OutDataTypeStr=Inherit: Same as input
  a(3)(2) : Gain  Gain=0.996999310040294295  ParamDataTypeStr=double  RndMeth=Nearest  SaturateOnIntegerOverflow=on  OutDataTypeStr=Inherit: Same as input
  a(3)(3) : Gain  Gain=0.991261883220059481  ParamDataTypeStr=double  RndMeth=Nearest  SaturateOnIntegerOverflow=on  OutDataTypeStr=Inherit: Same as input
  a(3)(4) : Gain  Gain=0.991734500200191382  ParamDataTypeStr=double  RndMeth=Nearest  SaturateOnIntegerOverflow=on  OutDataTypeStr=Inherit: Same as input
  a(3)(5) : Gain  Gain=0.988283107145958351  ParamDataTypeStr=double  RndMeth=Nearest  SaturateOnIntegerOverflow=on  OutDataTypeStr=Inherit: Same as input
  a(3)(6) : Gain  Gain=0.98851886923390353  ParamDataTypeStr=double  RndMeth=Nearest  SaturateOnIntegerOverflow=on  OutDataTypeStr=Inherit: Same as input
  s(1) : Gain  Gain=0.0249744654943331625  ParamDataTypeStr=double  RndMeth=Nearest  SaturateOnIntegerOverflow=on  OutDataTypeStr=Inherit: Same as input
  s(2) : Gain  Gain=0.0249744654943331625  ParamDataTypeStr=double  RndMeth=Nearest  SaturateOnIntegerOverflow=on  OutDataTypeStr=Inherit: Same as input
  s(3) : Gain  Gain=0.0186903150291075661  ParamDataTypeStr=double  RndMeth=Nearest  SaturateOnIntegerOverflow=on  OutDataTypeStr=Inherit: Same as input
  s(4) : Gain  Gain=0.0186903150291075661  ParamDataTypeStr=double  RndMeth=Nearest  SaturateOnIntegerOverflow=on  OutDataTypeStr=Inherit: Same as input
  s(5) : Gain  Gain=0.00882552998553024111  ParamDataTypeStr=double  RndMeth=Nearest  SaturateOnIntegerOverflow=on  OutDataTypeStr=Inherit: Same as input
  s(6) : Gain  Gain=0.00882552998553024111  ParamDataTypeStr=double  RndMeth=Nearest  SaturateOnIntegerOverflow=on  OutDataTypeStr=Inherit: Same as input
  s(7) : Gain  Gain=0.891250938133745563  ParamDataTypeStr=double  RndMeth=Nearest  SaturateOnIntegerOverflow=on  OutDataTypeStr=Inherit: Same as input
  Output : Outport
  wires:
  Input/1 -> s(1)/1
  s(1)/1 -> SumA21/1
  SumA21/1 -> SumA31/1
  SumA31/1 -> SumB31/1, Delay11/1
  SumB31/1 -> [Sect1]
  a(2)(1)/1 -> SumA21/2
  Delay11/1 -> a(2)(1)/1, Delay21/1
  a(3)(1)/1 -> SumA31/2
  Delay21/1 -> a(3)(1)/1, SumB31/2
  [Sect1] -> s(2)/1
  s(2)/1 -> SumA22/1
  SumA22/1 -> SumA32/1
  SumA32/1 -> SumB32/1, Delay12/1
  SumB32/1 -> [Sect2]
  a(2)(2)/1 -> SumA22/2
  Delay12/1 -> a(2)(2)/1, Delay22/1
  a(3)(2)/1 -> SumA32/2
  Delay22/1 -> a(3)(2)/1, SumB32/2
  [Sect2] -> s(3)/1
  s(3)/1 -> SumA23/1
  SumA23/1 -> SumA33/1
  SumA33/1 -> SumB33/1, Delay13/1
  SumB33/1 -> [Sect3]
  a(2)(3)/1 -> SumA23/2
  Delay13/1 -> a(2)(3)/1, Delay23/1
  a(3)(3)/1 -> SumA33/2
  Delay23/1 -> a(3)(3)/1, SumB33/2
  [Sect3] -> s(4)/1
  s(4)/1 -> SumA24/1
  SumA24/1 -> SumA34/1
  SumA34/1 -> SumB34/1, Delay14/1
  SumB34/1 -> [Sect4]
  a(2)(4)/1 -> SumA24/2
  Delay14/1 -> a(2)(4)/1, Delay24/1
  a(3)(4)/1 -> SumA34/2
  Delay24/1 -> a(3)(4)/1, SumB34/2
  [Sect4] -> s(5)/1
  s(5)/1 -> SumA25/1
  SumA25/1 -> SumA35/1
  SumA35/1 -> SumB35/1, Delay15/1
  SumB35/1 -> [Sect5]
  a(2)(5)/1 -> SumA25/2
  Delay15/1 -> a(2)(5)/1, Delay25/1
  a(3)(5)/1 -> SumA35/2
  Delay25/1 -> a(3)(5)/1, SumB35/2
  [Sect5] -> s(6)/1
  s(6)/1 -> SumA26/1
  SumA26/1 -> SumA36/1
  SumA36/1 -> SumB36/1, Delay16/1
  SumB36/1 -> s(7)/1
  a(2)(6)/1 -> SumA26/2
  Delay16/1 -> a(2)(6)/1, Delay26/1
  a(3)(6)/1 -> SumA36/2
  Delay26/1 -> a(3)(6)/1, SumB36/2
  s(7)/1 -> Output/1

== system Previous_Version_2016_b_All_BPF_with_IQ_Demodulation/23KHz DPA Demodulator ==
  note: "Imaginary"
  note: "Real"
  Output : Inport
  Delay : Delay  DelayLength=1  InitialCondition=0
  Delay1 : Delay  DelayLength=1  InitialCondition=0
  Divide : Product  Inputs=*/
  Gain1 : Gain  Gain=7.5/((0.000004)*(2*pi*1000))
  Gain2 : Gain  Gain=-1
  LPF_23080Hz_Elliptical_100dB_BW_2KHz_Order_1 : Subsystem  Tag=FilterWizardSubSystem
      settings: ErrorFcn=dspFilterRealizedInBasicElemsAlgLoopErrFcnCallback
  LPF_23080Hz_Elliptical_100dB_BW_2KHz_Order_10 : Subsystem  Tag=FilterWizardSubSystem
      settings: ErrorFcn=dspFilterRealizedInBasicElemsAlgLoopErrFcnCallback
  Product{5..10} (6 alike) : Product
  Scope : Scope
  Scope5 : Scope
  Scope6 : Scope
  Sine Wave : Sin  Frequency=2*pi*23080  Phase=+(pi/2)  Samples=250  SampleTime=1/250000
  Sine Wave1 : Sin  Frequency=2*pi*23080  SampleTime=1/250000
  Sum : Sum  Inputs=|++
  Sum1 : Sum  Inputs=|+-
  Trigonometric Function1 : Trigonometry  Operator=atan
  Out1 : Outport
  wires:
  LPF_23080Hz_Elliptical_100dB_BW_2KHz_Order_10/1(Output) -> Scope5/1, Product10/1, Product9/1, Delay1/1
  Delay/1 -> Product8/1, Product9/2
  Gain2/1 -> Product8/2, Product6/2, Delay/1
  Delay1/1 -> Product6/1, Product10/2
  Divide/1 -> Trigonometric Function1/1
  Gain1/1 -> Out1/1
  Product6/1 -> Sum1/1
  Sum/1 -> Divide/2
  Sum1/1 -> Divide/1
  Product5/1 -> LPF_23080Hz_Elliptical_100dB_BW_2KHz_Order_10/1(Input)
  Product8/1 -> Sum/2
  Product9/1 -> Sum1/2
  Sine Wave1/1 -> Product5/2
  Output/1 -> Product5/1, Product7/2, Scope/1
  LPF_23080Hz_Elliptical_100dB_BW_2KHz_Order_1/1(Output) -> Gain2/1, Scope6/1
  Product10/1 -> Sum/1
  Sine Wave/1 -> Product7/1
  Product7/1 -> LPF_23080Hz_Elliptical_100dB_BW_2KHz_Order_1/1(Input)
  Trigonometric Function1/1 -> Gain1/1

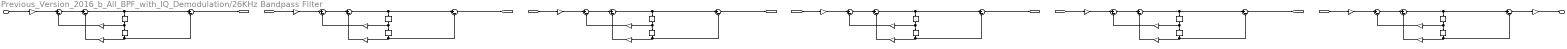
== system Previous_Version_2016_b_All_BPF_with_IQ_Demodulation/26KHz Bandpass Filter ==
  Input : Inport
  Delay{11..16,21..26} (12 alike) : Delay  DelayLength=1  InitialCondition=0
  SumA{21..26,31..36} (12 alike) : Sum  Inputs=|+-  RndMeth=Nearest  SaturateOnIntegerOverflow=on  OutDataTypeStr=Inherit: Same as first input
  SumB{31..36} (6 alike) : Sum  Inputs=|+-  RndMeth=Nearest  SaturateOnIntegerOverflow=on  OutDataTypeStr=Inherit: Same as first input
  a(2)(1) : Gain  Gain=-1.54863051875398416  ParamDataTypeStr=double  RndMeth=Nearest  SaturateOnIntegerOverflow=on  OutDataTypeStr=Inherit: Same as input
  a(2)(2) : Gain  Gain=-1.60977902978997767  ParamDataTypeStr=double  RndMeth=Nearest  SaturateOnIntegerOverflow=on  OutDataTypeStr=Inherit: Same as input
  a(2)(3) : Gain  Gain=-1.55298432204988468  ParamDataTypeStr=double  RndMeth=Nearest  SaturateOnIntegerOverflow=on  OutDataTypeStr=Inherit: Same as input
  a(2)(4) : Gain  Gain=-1.59782471963330908  ParamDataTypeStr=double  RndMeth=Nearest  SaturateOnIntegerOverflow=on  OutDataTypeStr=Inherit: Same as input
  a(2)(5) : Gain  Gain=-1.56519373811396223  ParamDataTypeStr=double  RndMeth=Nearest  SaturateOnIntegerOverflow=on  OutDataTypeStr=Inherit: Same as input
  a(2)(6) : Gain  Gain=-1.58162197849541331  ParamDataTypeStr=double  RndMeth=Nearest  SaturateOnIntegerOverflow=on  OutDataTypeStr=Inherit: Same as input
  a(3)(1) : Gain  Gain=0.996780024747651039  ParamDataTypeStr=double  RndMeth=Nearest  SaturateOnIntegerOverflow=on  OutDataTypeStr=Inherit: Same as input
  a(3)(2) : Gain  Gain=0.996981193126482701  ParamDataTypeStr=double  RndMeth=Nearest  SaturateOnIntegerOverflow=on  OutDataTypeStr=Inherit: Same as input
  a(3)(3) : Gain  Gain=0.991297958883154973  ParamDataTypeStr=double  RndMeth=Nearest  SaturateOnIntegerOverflow=on  OutDataTypeStr=Inherit: Same as input
  a(3)(4) : Gain  Gain=0.991698408650328656  ParamDataTypeStr=double  RndMeth=Nearest  SaturateOnIntegerOverflow=on  OutDataTypeStr=Inherit: Same as input
  a(3)(5) : Gain  Gain=0.988301115279193176  ParamDataTypeStr=double  RndMeth=Nearest  SaturateOnIntegerOverflow=on  OutDataTypeStr=Inherit: Same as input
  a(3)(6) : Gain  Gain=0.988500857132906363  ParamDataTypeStr=double  RndMeth=Nearest  SaturateOnIntegerOverflow=on  OutDataTypeStr=Inherit: Same as input
  s(1) : Gain  Gain=0.0249744654943332769  ParamDataTypeStr=double  RndMeth=Nearest  SaturateOnIntegerOverflow=on  OutDataTypeStr=Inherit: Same as input
  s(2) : Gain  Gain=0.0249744654943332769  ParamDataTypeStr=double  RndMeth=Nearest  SaturateOnIntegerOverflow=on  OutDataTypeStr=Inherit: Same as input
  s(3) : Gain  Gain=0.0186903150291076563  ParamDataTypeStr=double  RndMeth=Nearest  SaturateOnIntegerOverflow=on  OutDataTypeStr=Inherit: Same as input
  s(4) : Gain  Gain=0.0186903150291076563  ParamDataTypeStr=double  RndMeth=Nearest  SaturateOnIntegerOverflow=on  OutDataTypeStr=Inherit: Same as input
  s(5) : Gain  Gain=0.00882552998553028101  ParamDataTypeStr=double  RndMeth=Nearest  SaturateOnIntegerOverflow=on  OutDataTypeStr=Inherit: Same as input
  s(6) : Gain  Gain=0.00882552998553028101  ParamDataTypeStr=double  RndMeth=Nearest  SaturateOnIntegerOverflow=on  OutDataTypeStr=Inherit: Same as input
  s(7) : Gain  Gain=0.891250938133745563  ParamDataTypeStr=double  RndMeth=Nearest  SaturateOnIntegerOverflow=on  OutDataTypeStr=Inherit: Same as input
  Output : Outport
  wires:
  Input/1 -> s(1)/1
  s(1)/1 -> SumA21/1
  SumA21/1 -> SumA31/1
  SumA31/1 -> SumB31/1, Delay11/1
  SumB31/1 -> [Sect1]
  a(2)(1)/1 -> SumA21/2
  Delay11/1 -> a(2)(1)/1, Delay21/1
  a(3)(1)/1 -> SumA31/2
  Delay21/1 -> a(3)(1)/1, SumB31/2
  [Sect1] -> s(2)/1
  s(2)/1 -> SumA22/1
  SumA22/1 -> SumA32/1
  SumA32/1 -> SumB32/1, Delay12/1
  SumB32/1 -> [Sect2]
  a(2)(2)/1 -> SumA22/2
  Delay12/1 -> a(2)(2)/1, Delay22/1
  a(3)(2)/1 -> SumA32/2
  Delay22/1 -> a(3)(2)/1, SumB32/2
  [Sect2] -> s(3)/1
  s(3)/1 -> SumA23/1
  SumA23/1 -> SumA33/1
  SumA33/1 -> SumB33/1, Delay13/1
  SumB33/1 -> [Sect3]
  a(2)(3)/1 -> SumA23/2
  Delay13/1 -> a(2)(3)/1, Delay23/1
  a(3)(3)/1 -> SumA33/2
  Delay23/1 -> a(3)(3)/1, SumB33/2
  [Sect3] -> s(4)/1
  s(4)/1 -> SumA24/1
  SumA24/1 -> SumA34/1
  SumA34/1 -> SumB34/1, Delay14/1
  SumB34/1 -> [Sect4]
  a(2)(4)/1 -> SumA24/2
  Delay14/1 -> a(2)(4)/1, Delay24/1
  a(3)(4)/1 -> SumA34/2
  Delay24/1 -> a(3)(4)/1, SumB34/2
  [Sect4] -> s(5)/1
  s(5)/1 -> SumA25/1
  SumA25/1 -> SumA35/1
  SumA35/1 -> SumB35/1, Delay15/1
  SumB35/1 -> [Sect5]
  a(2)(5)/1 -> SumA25/2
  Delay15/1 -> a(2)(5)/1, Delay25/1
  a(3)(5)/1 -> SumA35/2
  Delay25/1 -> a(3)(5)/1, SumB35/2
  [Sect5] -> s(6)/1
  s(6)/1 -> SumA26/1
  SumA26/1 -> SumA36/1
  SumA36/1 -> SumB36/1, Delay16/1
  SumB36/1 -> s(7)/1
  a(2)(6)/1 -> SumA26/2
  Delay16/1 -> a(2)(6)/1, Delay26/1
  a(3)(6)/1 -> SumA36/2
  Delay26/1 -> a(3)(6)/1, SumB36/2
  s(7)/1 -> Output/1

== system Previous_Version_2016_b_All_BPF_with_IQ_Demodulation/26KHz DPA Demodulator ==
  note: "Imaginary"
  note: "Real"
  Output : Inport
  Delay : Delay  DelayLength=1  InitialCondition=0
  Delay1 : Delay  DelayLength=1  InitialCondition=0
  Divide : Product  Inputs=*/
  Gain1 : Gain  Gain=7.5/((0.000004)*(2*pi*1000))
  Gain2 : Gain  Gain=-1
  LPF_26190Hz_Elliptical_100dB_BW_2KHz_Order_1 : Subsystem  Tag=FilterWizardSubSystem
      settings: ErrorFcn=dspFilterRealizedInBasicElemsAlgLoopErrFcnCallback
  LPF_26190Hz_Elliptical_100dB_BW_2KHz_Order_10 : Subsystem  Tag=FilterWizardSubSystem
      settings: ErrorFcn=dspFilterRealizedInBasicElemsAlgLoopErrFcnCallback
  Product{5..10} (6 alike) : Product
  Scope : Scope
  Scope5 : Scope
  Scope6 : Scope
  Sine Wave : Sin  Frequency=2*pi*26190  Phase=+(pi/2)  Samples=250  SampleTime=1/250000
  Sine Wave1 : Sin  Frequency=2*pi*26190  SampleTime=1/250000
  Sum : Sum  Inputs=|++
  Sum1 : Sum  Inputs=|+-
  Trigonometric Function1 : Trigonometry  Operator=atan
  Out1 : Outport
  wires:
  LPF_26190Hz_Elliptical_100dB_BW_2KHz_Order_10/1(Output) -> Scope5/1, Product10/1, Product9/1, Delay1/1
  Delay/1 -> Product8/1, Product9/2
  Gain2/1 -> Product8/2, Product6/2, Delay/1
  Delay1/1 -> Product6/1, Product10/2
  Divide/1 -> Trigonometric Function1/1
  Gain1/1 -> Out1/1
  Product6/1 -> Sum1/1
  Sum/1 -> Divide/2
  Sum1/1 -> Divide/1
  Product5/1 -> LPF_26190Hz_Elliptical_100dB_BW_2KHz_Order_10/1(Input)
  Product8/1 -> Sum/2
  Product9/1 -> Sum1/2
  Sine Wave1/1 -> Product5/2
  Output/1 -> Product5/1, Product7/2, Scope/1
  LPF_26190Hz_Elliptical_100dB_BW_2KHz_Order_1/1(Output) -> Gain2/1, Scope6/1
  Product10/1 -> Sum/1
  Sine Wave/1 -> Product7/1
  Product7/1 -> LPF_26190Hz_Elliptical_100dB_BW_2KHz_Order_1/1(Input)
  Trigonometric Function1/1 -> Gain1/1

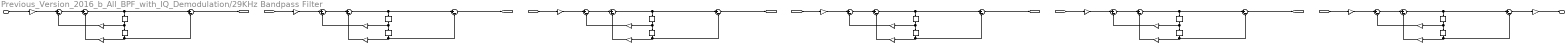
== system Previous_Version_2016_b_All_BPF_with_IQ_Demodulation/29KHz Bandpass Filter ==
  Input : Inport
  Delay{11..16,21..26} (12 alike) : Delay  DelayLength=1  InitialCondition=0
  SumA{21..26,31..36} (12 alike) : Sum  Inputs=|+-  RndMeth=Nearest  SaturateOnIntegerOverflow=on  OutDataTypeStr=Inherit: Same as first input
  SumB{31..36} (6 alike) : Sum  Inputs=|+-  RndMeth=Nearest  SaturateOnIntegerOverflow=on  OutDataTypeStr=Inherit: Same as first input
  a(2)(1) : Gain  Gain=-1.45411391212130514  ParamDataTypeStr=double  RndMeth=Nearest  SaturateOnIntegerOverflow=on  OutDataTypeStr=Inherit: Same as input
  a(2)(2) : Gain  Gain=-1.52073981225900523  ParamDataTypeStr=double  RndMeth=Nearest  SaturateOnIntegerOverflow=on  OutDataTypeStr=Inherit: Same as input
  a(2)(3) : Gain  Gain=-1.45944525212328591  ParamDataTypeStr=double  RndMeth=Nearest  SaturateOnIntegerOverflow=on  OutDataTypeStr=Inherit: Same as input
  a(2)(4) : Gain  Gain=-1.50824968053149533  ParamDataTypeStr=double  RndMeth=Nearest  SaturateOnIntegerOverflow=on  OutDataTypeStr=Inherit: Same as input
  a(2)(5) : Gain  Gain=-1.4730318681214829  ParamDataTypeStr=double  RndMeth=Nearest  SaturateOnIntegerOverflow=on  OutDataTypeStr=Inherit: Same as input
  a(2)(6) : Gain  Gain=-1.49090181768233965  ParamDataTypeStr=double  RndMeth=Nearest  SaturateOnIntegerOverflow=on  OutDataTypeStr=Inherit: Same as input
  a(3)(1) : Gain  Gain=0.996793715113723278  ParamDataTypeStr=double  RndMeth=Nearest  SaturateOnIntegerOverflow=on  OutDataTypeStr=Inherit: Same as input
  a(3)(2) : Gain  Gain=0.996967500185515831  ParamDataTypeStr=double  RndMeth=Nearest  SaturateOnIntegerOverflow=on  OutDataTypeStr=Inherit: Same as input
  a(3)(3) : Gain  Gain=0.991325219830234139  ParamDataTypeStr=double  RndMeth=Nearest  SaturateOnIntegerOverflow=on  OutDataTypeStr=Inherit: Same as input
  a(3)(4) : Gain  Gain=0.991671137440741202  ParamDataTypeStr=double  RndMeth=Nearest  SaturateOnIntegerOverflow=on  OutDataTypeStr=Inherit: Same as input
  a(3)(5) : Gain  Gain=0.988314719744223247  ParamDataTypeStr=double  RndMeth=Nearest  SaturateOnIntegerOverflow=on  OutDataTypeStr=Inherit: Same as input
  a(3)(6) : Gain  Gain=0.988487250105640092  ParamDataTypeStr=double  RndMeth=Nearest  SaturateOnIntegerOverflow=on  OutDataTypeStr=Inherit: Same as input
  s(1) : Gain  Gain=0.0249744654943332006  ParamDataTypeStr=double  RndMeth=Nearest  SaturateOnIntegerOverflow=on  OutDataTypeStr=Inherit: Same as input
  s(2) : Gain  Gain=0.0249744654943332006  ParamDataTypeStr=double  RndMeth=Nearest  SaturateOnIntegerOverflow=on  OutDataTypeStr=Inherit: Same as input
  s(3) : Gain  Gain=0.0186903150291075973  ParamDataTypeStr=double  RndMeth=Nearest  SaturateOnIntegerOverflow=on  OutDataTypeStr=Inherit: Same as input
  s(4) : Gain  Gain=0.0186903150291075973  ParamDataTypeStr=double  RndMeth=Nearest  SaturateOnIntegerOverflow=on  OutDataTypeStr=Inherit: Same as input
  s(5) : Gain  Gain=0.00882552998553025499  ParamDataTypeStr=double  RndMeth=Nearest  SaturateOnIntegerOverflow=on  OutDataTypeStr=Inherit: Same as input
  s(6) : Gain  Gain=0.00882552998553025499  ParamDataTypeStr=double  RndMeth=Nearest  SaturateOnIntegerOverflow=on  OutDataTypeStr=Inherit: Same as input
  s(7) : Gain  Gain=0.891250938133745563  ParamDataTypeStr=double  RndMeth=Nearest  SaturateOnIntegerOverflow=on  OutDataTypeStr=Inherit: Same as input
  Output : Outport
  wires:
  Input/1 -> s(1)/1
  s(1)/1 -> SumA21/1
  SumA21/1 -> SumA31/1
  SumA31/1 -> SumB31/1, Delay11/1
  SumB31/1 -> [Sect1]
  a(2)(1)/1 -> SumA21/2
  Delay11/1 -> a(2)(1)/1, Delay21/1
  a(3)(1)/1 -> SumA31/2
  Delay21/1 -> a(3)(1)/1, SumB31/2
  [Sect1] -> s(2)/1
  s(2)/1 -> SumA22/1
  SumA22/1 -> SumA32/1
  SumA32/1 -> SumB32/1, Delay12/1
  SumB32/1 -> [Sect2]
  a(2)(2)/1 -> SumA22/2
  Delay12/1 -> a(2)(2)/1, Delay22/1
  a(3)(2)/1 -> SumA32/2
  Delay22/1 -> a(3)(2)/1, SumB32/2
  [Sect2] -> s(3)/1
  s(3)/1 -> SumA23/1
  SumA23/1 -> SumA33/1
  SumA33/1 -> SumB33/1, Delay13/1
  SumB33/1 -> [Sect3]
  a(2)(3)/1 -> SumA23/2
  Delay13/1 -> a(2)(3)/1, Delay23/1
  a(3)(3)/1 -> SumA33/2
  Delay23/1 -> a(3)(3)/1, SumB33/2
  [Sect3] -> s(4)/1
  s(4)/1 -> SumA24/1
  SumA24/1 -> SumA34/1
  SumA34/1 -> SumB34/1, Delay14/1
  SumB34/1 -> [Sect4]
  a(2)(4)/1 -> SumA24/2
  Delay14/1 -> a(2)(4)/1, Delay24/1
  a(3)(4)/1 -> SumA34/2
  Delay24/1 -> a(3)(4)/1, SumB34/2
  [Sect4] -> s(5)/1
  s(5)/1 -> SumA25/1
  SumA25/1 -> SumA35/1
  SumA35/1 -> SumB35/1, Delay15/1
  SumB35/1 -> [Sect5]
  a(2)(5)/1 -> SumA25/2
  Delay15/1 -> a(2)(5)/1, Delay25/1
  a(3)(5)/1 -> SumA35/2
  Delay25/1 -> a(3)(5)/1, SumB35/2
  [Sect5] -> s(6)/1
  s(6)/1 -> SumA26/1
  SumA26/1 -> SumA36/1
  SumA36/1 -> SumB36/1, Delay16/1
  SumB36/1 -> s(7)/1
  a(2)(6)/1 -> SumA26/2
  Delay16/1 -> a(2)(6)/1, Delay26/1
  a(3)(6)/1 -> SumA36/2
  Delay26/1 -> a(3)(6)/1, SumB36/2
  s(7)/1 -> Output/1
